simulink model "experiment_cl"  (R2017a)
settings: Solver=VariableStepAuto  StartTime=0.0  StopTime=30  RelTol=1e-3
settings Model: Creator=GUJINGQIANG  LastModifiedBy=Mr.li

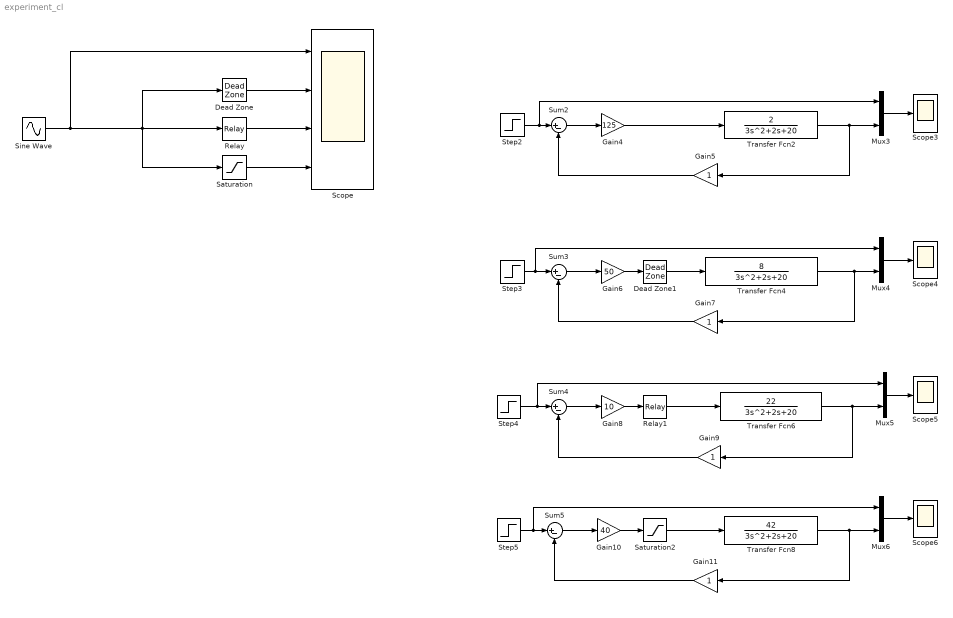
== system experiment_cl ==
  Dead Zone : DeadZone  SaturateOnIntegerOverflow=on
  Dead Zone1 : DeadZone  SaturateOnIntegerOverflow=on
  Gain10 : Gain  Gain=40
  Gain{5,7,9,11} (4 alike) : Gain
  Gain4 : Gain  Gain=125
  Gain6 : Gain  Gain=50
  Gain8 : Gain  Gain=10
  Mux{3..6} (4 alike) : Mux  Inputs=2
  Relay : Relay
  Relay1 : Relay
  Saturation : Saturate
  Saturation2 : Saturate
  Scope : Scope  NumInputPorts=4
  Scope{3..6} (4 alike) : Scope
  Sine Wave : Sin  SampleTime=0
  Step{2..5} (4 alike) : Step  SampleTime=0
  Sum{2..5} (4 alike) : Sum  Inputs=|+-
  Transfer Fcn2 : TransferFcn  Numerator=[2]  Denominator=[3 2 20]
  Transfer Fcn4 : TransferFcn  Numerator=8  Denominator=[3 2 20]
  Transfer Fcn6 : TransferFcn  Numerator=22  Denominator=[3 2 20]
  Transfer Fcn8 : TransferFcn  Numerator=42  Denominator=[3 2 20]
  wires:
  Sine Wave/1 -> Scope/1, Saturation/1, Dead Zone/1, Relay/1
  Saturation/1 -> Scope/4
  Relay/1 -> Scope/3
  Dead Zone/1 -> Scope/2
  Step2/1 -> Mux3/1, Sum2/1
  Sum2/1 -> Gain4/1
  Mux3/1 -> Scope3/1
  Gain5/1 -> Sum2/2
  Transfer Fcn2/1 -> Gain5/1, Mux3/2
  Gain4/1 -> Transfer Fcn2/1
  Step3/1 -> Mux4/1, Sum3/1
  Sum3/1 -> Gain6/1
  Mux4/1 -> Scope4/1
  Gain7/1 -> Sum3/2
  Transfer Fcn4/1 -> Gain7/1, Mux4/2
  Mux5/1 -> Scope5/1
  Transfer Fcn6/1 -> Gain9/1, Mux5/2
  Relay1/1 -> Transfer Fcn6/1
  Step5/1 -> Mux6/1, Sum5/1
  Sum5/1 -> Gain10/1
  Mux6/1 -> Scope6/1
  Gain11/1 -> Sum5/2
  Transfer Fcn8/1 -> Gain11/1, Mux6/2
  Saturation2/1 -> Transfer Fcn8/1
  Gain6/1 -> Dead Zone1/1
  Dead Zone1/1 -> Transfer Fcn4/1
  Gain8/1 -> Relay1/1
  Gain10/1 -> Saturation2/1
  Step4/1 -> Mux5/1, Sum4/1
  Sum4/1 -> Gain8/1
  Gain9/1 -> Sum4/2
